simulink model "Amortiguador"  (R2022b)
settings: Solver=VariableStepAuto  StartTime=0.0  StopTime=10.0  RelTol=1e-3
values from neighbouring files (symbols this model uses):
  b1 = 1000    [Amortiguadorp.m]    (also in IntegracionAutomovil.m)
  k1 = 16182    [Amortiguadorp.m]    (also in IntegracionAutomovil.m)
  k2 = 19000    [Amortiguadorp.m]    (also in IntegracionAutomovil.m)
  m1 = 290    [Amortiguadorp.m]    (also in IntegracionAutomovil.m)
  m2 = 59    [Amortiguadorp.m]    (also in IntegracionAutomovil.m)
settings Model: Creator=nemesis  LastModifiedBy=nemesis

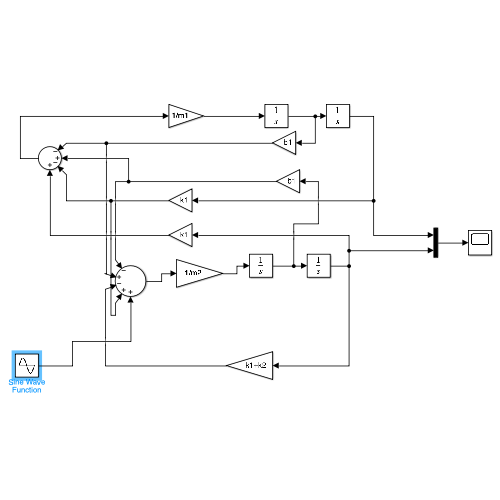
[thumbnail: Simulink's stored preview of the top-level diagram]
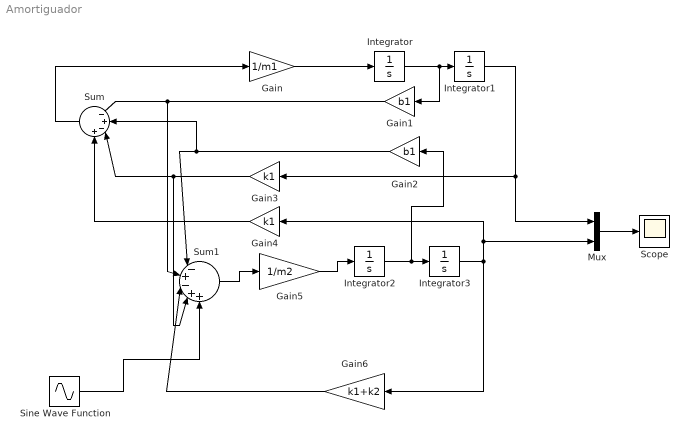
== system Amortiguador ==
  Gain : Gain  Gain=1/m1
  Gain1 : Gain  Gain=b1
  Gain2 : Gain  Gain=b1
  Gain3 : Gain  Gain=k1
  Gain4 : Gain  Gain=k1
  Gain5 : Gain  Gain=1/m2
  Gain6 : Gain  Gain=k1+k2
  Integrator{,1..3} (4 alike) : Integrator
  Mux : Mux  Inputs=2
  Scope : Scope
  Sine Wave Function : Sin  Amplitude=0.05*k2  Frequency=20*pi  SampleTime=0
  Sum : Sum  Inputs=|-+-+
  Sum1 : Sum  Inputs=|-+-++
  wires:
  Integrator/1 -> Gain1/1, Integrator1/1
  Integrator2/1 -> Gain2/1, Integrator3/1
  Gain1/1 -> Sum1/2, Sum/1
  Gain2/1 -> Sum1/1, Sum/2
  Integrator1/1 -> Mux/1, Gain3/1
  Gain3/1 -> Sum1/4, Sum/3
  Integrator3/1 -> Mux/2, Gain4/1, Gain6/1
  Gain4/1 -> Sum/4
  Sum/1 -> Gain/1
  Gain/1 -> Integrator/1
  Gain6/1 -> Sum1/3
  Sum1/1 -> Gain5/1
  Gain5/1 -> Integrator2/1
  Sine Wave Function/1 -> Sum1/5
  Mux/1 -> Scope/1
